simulink model "dynamical_model_extended"  (R2017b)
settings: Solver=ode4  StartTime=0.0  StopTime=3  FixedStep=dt  RelTol=1e-3
undefined symbols (not defined in the file or in its folder): alpha0, c1, c2, c3, d0, dq_0, g, m, p_true, q_0, r
libraries: dspinverses x2
(part 3 of 3)

== matlab function dynamical_model_extended/soft robotic manipulator dynamical model/Inertia matrix  ==
  data: q input; y output; m parameter; r parameter
function y = fcn(q,m,r)

l1 = q(1);
kappa_x1 = q(2);
kappa_y1 = q(3);

M = zeros(3,3);

% M(1,1) = (2.0*kappa_x1^2*l1*m*(kappa_x1^2 + kappa_y1^2)^(3/2) - 4.0*kappa_x1^4*m*sin(l1*(kappa_x1^2 + kappa_y1^2)^(1/2)) + 2.0*kappa_x1^4*l1*m*(kappa_x1^2 + kappa_y1^2)^(1/2) + 0.66666666666666666666666666666667*kappa_y1^4*l1^3*m*(kappa_x1^2 + kappa_y1^2)^(3/2) - 4.0*kappa_x1^2*kappa_y1^2*m*sin(l1*(kappa_x1^2 + kappa_y1^2)^(1/2)) + 2.0*kappa_x1^2*kappa_y1^2*l1*m*(kappa_x1^2 + kappa_y1^2)^(1/2) + (2/3)*kappa_x1^2*kappa_y1^2*l1^3*m*(kappa_x1^2 + kappa_y1^2)^(3/2))/(l1*(kappa_x1^2 + kappa_y1^2)^(7/2));
% M(1,2) =  -(1.0*kappa_x1*m*((kappa_x1^2 + kappa_y1^2)/kappa_x1^2)^(1/2)*(2.0*cos(l1*(kappa_x1^2 + kappa_y1^2)^(1/2))*(kappa_x1^2 + kappa_y1^2)^(1/2) - 2.0*(kappa_x1^2 + kappa_y1^2)^(1/2) + 2.0*kappa_x1^2*l1*sin(l1*(kappa_x1^2 + kappa_y1^2)^(1/2)) + 2.0*kappa_y1^2*l1*sin(l1*(kappa_x1^2 + kappa_y1^2)^(1/2)) - kappa_x1^2*l1^2*(kappa_x1^2 + kappa_y1^2)^(1/2) - kappa_y1^2*l1^2*(kappa_x1^2 + kappa_y1^2)^(1/2)))/(l1*(kappa_x1^2 + kappa_y1^2)^3);
% M(1,3) = 0;
% 
% M(2,1) = M(1,2);
% M(2,2) = (1.6e34*kappa_x1^4*l1*m + 1.2e34*kappa_y1^4*l1*m + 2.6666666666666666666666666666667e33*kappa_x1^6*l1^3*m + 2.6666666666666666666666666666667e33*kappa_x1^2*kappa_y1^4*l1^3*m + 5.3333333333333333333333333333333e33*kappa_x1^4*kappa_y1^2*l1^3*m + 666666666666666666666666666666677.0*kappa_x1^8*l1^3*m*r^2 - 3.2e34*kappa_x1^2*m*sin(l1*(kappa_x1^2 + kappa_y1^2)^(1/2))*(kappa_x1^2 + kappa_y1^2)^(1/2) - 1.6e34*kappa_y1^2*m*sin(l1*(kappa_x1^2 + kappa_y1^2)^(1/2))*(kappa_x1^2 + kappa_y1^2)^(1/2) + 1.6e34*kappa_x1^4*l1*m*cos(l1*(kappa_x1^2 + kappa_y1^2)^(1/2)) + 2.0e33*kappa_y1^2*m*sin(2.0*l1*(kappa_x1^2 + kappa_y1^2)^(1/2))*(kappa_x1^2 + kappa_y1^2)^(1/2) + 2.8e34*kappa_x1^2*kappa_y1^2*l1*m + 7.0e33*kappa_y1^6*l1*m*r^2 - 8.0e33*kappa_y1^2*m*r^2*sin(l1*(kappa_x1^2 + kappa_y1^2)^(1/2))*(kappa_x1^2 + kappa_y1^2)^(3/2) + 1.6e34*kappa_x1^2*kappa_y1^2*l1*m*cos(l1*(kappa_x1^2 + kappa_y1^2)^(1/2)) + 1.0e33*kappa_y1^2*m*r^2*sin(2.0*l1*(kappa_x1^2 + kappa_y1^2)^(1/2))*(kappa_x1^2 + kappa_y1^2)^(3/2) - 500000000000000000000000000000000.0*kappa_y1^4*m*r^2*sin(2.0*l1*(kappa_x1^2 + kappa_y1^2)^(1/2))*(kappa_x1^2 + kappa_y1^2)^(1/2) + 1.5e34*kappa_x1^2*kappa_y1^4*l1*m*r^2 + 8.0e33*kappa_x1^4*kappa_y1^2*l1*m*r^2 + 1.3333333333333333333333333333333e33*kappa_x1^2*kappa_y1^6*l1^3*m*r^2 + 3.3333333333333333333333333333333e33*kappa_x1^4*kappa_y1^4*l1^3*m*r^2 + 2.6666666666666666666666666666667e33*kappa_x1^6*kappa_y1^2*l1^3*m*r^2 - 4.0e33*kappa_x1^2*kappa_y1^2*m*r^2*sin(l1*(kappa_x1^2 + kappa_y1^2)^(1/2))*(kappa_x1^2 + kappa_y1^2)^(1/2) + 4.0e33*kappa_x1^2*kappa_y1^4*l1*m*r^2*cos(l1*(kappa_x1^2 + kappa_y1^2)^(1/2)) + 4.0e33*kappa_x1^4*kappa_y1^2*l1*m*r^2*cos(l1*(kappa_x1^2 + kappa_y1^2)^(1/2)) - 1.0e33*kappa_x1^2*kappa_y1^2*m*r^2*sin(2.0*l1*(kappa_x1^2 + kappa_y1^2)^(1/2))*(kappa_x1^2 + kappa_y1^2)^(1/2))/(4000000000000000000000000000000000*l1*(kappa_x1^2 + kappa_y1^2)^4);
% M(2,3) = (kappa_x1*kappa_y1*m*(1.0e33*kappa_x1^2*l1 - 500000000000000000000000000000000.0*sin(2.0*l1*(kappa_x1^2 + kappa_y1^2)^(1/2))*(kappa_x1^2 + kappa_y1^2)^(1/2) - 4.0e33*sin(l1*(kappa_x1^2 + kappa_y1^2)^(1/2))*(kappa_x1^2 + kappa_y1^2)^(1/2) + 1.0e33*kappa_y1^2*l1 + 666666666666666666666666666666677.0*kappa_x1^4*l1^3 + 666666666666666666666666666666677.0*kappa_y1^4*l1^3 + 2.0e33*r^2*sin(l1*(kappa_x1^2 + kappa_y1^2)^(1/2))*(kappa_x1^2 + kappa_y1^2)^(3/2) + 4.0e33*kappa_x1^2*l1*cos(l1*(kappa_x1^2 + kappa_y1^2)^(1/2)) + 4.0e33*kappa_y1^2*l1*cos(l1*(kappa_x1^2 + kappa_y1^2)^(1/2)) - 250000000000000000000000000000000.0*r^2*sin(2.0*l1*(kappa_x1^2 + kappa_y1^2)^(1/2))*(kappa_x1^2 + kappa_y1^2)^(3/2) - 2.0e33*kappa_x1^4*l1*r^2 - 1.75e33*kappa_y1^4*l1*r^2 + 1.3333333333333333333333333333333e33*kappa_x1^2*kappa_y1^2*l1^3 + 166666666666666666666666666666677.0*kappa_x1^6*l1^3*r^2 + 333333333333333333333333333333333.0*kappa_y1^6*l1^3*r^2 + 250000000000000000000000000000000.0*kappa_x1^2*r^2*sin(2.0*l1*(kappa_x1^2 + kappa_y1^2)^(1/2))*(kappa_x1^2 + kappa_y1^2)^(1/2) + 125000000000000000000000000000000.0*kappa_y1^2*r^2*sin(2.0*l1*(kappa_x1^2 + kappa_y1^2)^(1/2))*(kappa_x1^2 + kappa_y1^2)^(1/2) - 3.75e33*kappa_x1^2*kappa_y1^2*l1*r^2 + 833333333333333333333333333333333.0*kappa_x1^2*kappa_y1^4*l1^3*r^2 + 666666666666666666666666666666677.0*kappa_x1^4*kappa_y1^2*l1^3*r^2 + 500000000000000000000000000000000.0*kappa_x1^2*r^2*sin(l1*(kappa_x1^2 + kappa_y1^2)^(1/2))*(kappa_x1^2 + kappa_y1^2)^(1/2) - 500000000000000000000000000000000.0*kappa_y1^2*r^2*sin(l1*(kappa_x1^2 + kappa_y1^2)^(1/2))*(kappa_x1^2 + kappa_y1^2)^(1/2) - 500000000000000000000000000000000.0*kappa_x1^4*l1*r^2*cos(l1*(kappa_x1^2 + kappa_y1^2)^(1/2)) + 500000000000000000000000000000000.0*kappa_y1^4*l1*r^2*cos(l1*(kappa_x1^2 + kappa_y1^2)^(1/2))))/(1000000000000000000000000000000000*l1*(kappa_x1^2 + kappa_y1^2)^4);
% 
% M(3,1) = 0;
% M(3,2) = M(2,3);
% M(3,3) = (1.2e34*kappa_x1^4*l1*m + 1.6e34*kappa_y1^4*l1*m + 2.6666666666666666666666666666667e33*kappa_y1^6*l1^3*m + 5.3333333333333333333333333333333e33*kappa_x1^2*kappa_y1^4*l1^3*m + 2.6666666666666666666666666666667e33*kappa_x1^4*kappa_y1^2*l1^3*m + 1.3333333333333333333333333333333e33*kappa_y1^8*l1^3*m*r^2 - 1.6e34*kappa_x1^2*m*sin(l1*(kappa_x1^2 + kappa_y1^2)^(1/2))*(kappa_x1^2 + kappa_y1^2)^(1/2) - 3.2e34*kappa_y1^2*m*sin(l1*(kappa_x1^2 + kappa_y1^2)^(1/2))*(kappa_x1^2 + kappa_y1^2)^(1/2) + 1.6e34*kappa_y1^4*l1*m*cos(l1*(kappa_x1^2 + kappa_y1^2)^(1/2)) + 2.0e33*kappa_x1^2*m*sin(2.0*l1*(kappa_x1^2 + kappa_y1^2)^(1/2))*(kappa_x1^2 + kappa_y1^2)^(1/2) + 2.8e34*kappa_x1^2*kappa_y1^2*l1*m + 8.0e33*kappa_x1^6*l1*m*r^2 - 8.0e33*kappa_x1^2*m*r^2*sin(l1*(kappa_x1^2 + kappa_y1^2)^(1/2))*(kappa_x1^2 + kappa_y1^2)^(3/2) + 1.6e34*kappa_x1^2*kappa_y1^2*l1*m*cos(l1*(kappa_x1^2 + kappa_y1^2)^(1/2)) + 1.0e33*kappa_x1^2*m*r^2*sin(2.0*l1*(kappa_x1^2 + kappa_y1^2)^(1/2))*(kappa_x1^2 + kappa_y1^2)^(3/2) - 1.0e33*kappa_x1^4*m*r^2*sin(2.0*l1*(kappa_x1^2 + kappa_y1^2)^(1/2))*(kappa_x1^2 + kappa_y1^2)^(1/2) + 7.0e33*kappa_x1^2*kappa_y1^4*l1*m*r^2 + 1.5e34*kappa_x1^4*kappa_y1^2*l1*m*r^2 + 3.3333333333333333333333333333333e33*kappa_x1^2*kappa_y1^6*l1^3*m*r^2 + 2.6666666666666666666666666666667e33*kappa_x1^4*kappa_y1^4*l1^3*m*r^2 + 666666666666666666666666666666677.0*kappa_x1^6*kappa_y1^2*l1^3*m*r^2 + 4.0e33*kappa_x1^2*kappa_y1^2*m*r^2*sin(l1*(kappa_x1^2 + kappa_y1^2)^(1/2))*(kappa_x1^2 + kappa_y1^2)^(1/2) - 4.0e33*kappa_x1^2*kappa_y1^4*l1*m*r^2*cos(l1*(kappa_x1^2 + kappa_y1^2)^(1/2)) - 4.0e33*kappa_x1^4*kappa_y1^2*l1*m*r^2*cos(l1*(kappa_x1^2 + kappa_y1^2)^(1/2)) - 500000000000000000000000000000000.0*kappa_x1^2*kappa_y1^2*m*r^2*sin(2.0*l1*(kappa_x1^2 + kappa_y1^2)^(1/2))*(kappa_x1^2 + kappa_y1^2)^(1/2))/(4000000000000000000000000000000000*l1*(kappa_x1^2 + kappa_y1^2)^4);
%  
%  
M(1,1) = (m*(l1*(kappa_x1^2 + kappa_y1^2)^(3/2) - 4.0*kappa_x1^2*sin(l1*(kappa_x1^2 + kappa_y1^2)^(1/2)) - 4.0*kappa_y1^2*sin(l1*(kappa_x1^2 + kappa_y1^2)^(1/2)) + 3.0*kappa_x1^2*l1*(kappa_x1^2 + kappa_y1^2)^(1/2) + 3.0*kappa_y1^2*l1*(kappa_x1^2 + kappa_y1^2)^(1/2)))/(l1*(kappa_x1^2 + kappa_y1^2)^(5/2));
M(1,2) = -(2*kappa_x1*m*(2.0*l1*(kappa_x1^2 + kappa_y1^2)^(1/2) - 3.0*sin(l1*(kappa_x1^2 + kappa_y1^2)^(1/2)) + l1*cos(l1*(kappa_x1^2 + kappa_y1^2)^(1/2))*(kappa_x1^2 + kappa_y1^2)^(1/2)))/(l1*(kappa_x1^2 + kappa_y1^2)^(5/2));
M(1,3) = -(2*kappa_y1*m*(2.0*l1*(kappa_x1^2 + kappa_y1^2)^(1/2) - 3.0*sin(l1*(kappa_x1^2 + kappa_y1^2)^(1/2)) + l1*cos(l1*(kappa_x1^2 + kappa_y1^2)^(1/2))*(kappa_x1^2 + kappa_y1^2)^(1/2)))/(l1*(kappa_x1^2 + kappa_y1^2)^(5/2));

M(2,1) = -(2*kappa_x1*m*(2.0*l1*(kappa_x1^2 + kappa_y1^2)^(1/2) - 3.0*sin(l1*(kappa_x1^2 + kappa_y1^2)^(1/2)) + l1*cos(l1*(kappa_x1^2 + kappa_y1^2)^(1/2))*(kappa_x1^2 + kappa_y1^2)^(1/2)))/(l1*(kappa_x1^2 + kappa_y1^2)^(5/2));
M(2,2) = (0.5*kappa_y1^2*m*sin(2.0*l1*(kappa_x1^2 + kappa_y1^2)^(1/2)) - 4.0*kappa_y1^2*m*sin(l1*(kappa_x1^2 + kappa_y1^2)^(1/2)) - 8.0*kappa_x1^2*m*sin(l1*(kappa_x1^2 + kappa_y1^2)^(1/2)) + 3.0*l1*m*(kappa_x1^2 + kappa_y1^2)^(3/2) + 0.125*kappa_y1^4*m*r^2*sin(2.0*l1*(kappa_x1^2 + kappa_y1^2)^(1/2)) + kappa_x1^2*l1*m*(kappa_x1^2 + kappa_y1^2)^(1/2) + 0.66666666666666666666666666666667*kappa_x1^2*l1^3*m*(kappa_x1^2 + kappa_y1^2)^(3/2) - 2.0*kappa_y1^4*m*r^2*sin(l1*(kappa_x1^2 + kappa_y1^2)^(1/2)) + 0.125*kappa_x1^2*kappa_y1^2*m*r^2*sin(2.0*l1*(kappa_x1^2 + kappa_y1^2)^(1/2)) + 1.5*kappa_y1^2*l1*m*r^2*(kappa_x1^2 + kappa_y1^2)^(3/2) + 0.25*kappa_y1^4*l1*m*r^2*(kappa_x1^2 + kappa_y1^2)^(1/2) + 0.16666666666666666666666666666667*kappa_x1^4*l1^3*m*r^2*(kappa_x1^2 + kappa_y1^2)^(3/2) - 2.0*kappa_x1^2*kappa_y1^2*m*r^2*sin(l1*(kappa_x1^2 + kappa_y1^2)^(1/2)) + 4.0*kappa_x1^2*l1*m*cos(l1*(kappa_x1^2 + kappa_y1^2)^(1/2))*(kappa_x1^2 + kappa_y1^2)^(1/2) + 0.16666666666666666666666666666667*kappa_x1^2*kappa_y1^2*l1^3*m*r^2*(kappa_x1^2 + kappa_y1^2)^(3/2) + 0.25*kappa_x1^2*kappa_y1^2*l1*m*r^2*(kappa_x1^2 + kappa_y1^2)^(1/2))/(l1*(kappa_x1^2 + kappa_y1^2)^(7/2));
M(2,3) = -(2.5e-34*kappa_x1*kappa_y1*m*(1.6e34*sin(l1*(kappa_x1^2 + kappa_y1^2)^(1/2)) + 2.0e33*sin(2.0*l1*(kappa_x1^2 + kappa_y1^2)^(1/2)) - 4.0e33*l1*(kappa_x1^2 + kappa_y1^2)^(1/2) - 2.6666666666666666666666666666667e33*l1^3*(kappa_x1^2 + kappa_y1^2)^(3/2) - 8.0e33*kappa_x1^2*r^2*sin(l1*(kappa_x1^2 + kappa_y1^2)^(1/2)) - 8.0e33*kappa_y1^2*r^2*sin(l1*(kappa_x1^2 + kappa_y1^2)^(1/2)) - 1.6e34*l1*cos(l1*(kappa_x1^2 + kappa_y1^2)^(1/2))*(kappa_x1^2 + kappa_y1^2)^(1/2) + 500000000000000000000000000000000.0*kappa_x1^2*r^2*sin(2.0*l1*(kappa_x1^2 + kappa_y1^2)^(1/2)) + 500000000000000000000000000000000.0*kappa_y1^2*r^2*sin(2.0*l1*(kappa_x1^2 + kappa_y1^2)^(1/2)) + 6.0e33*l1*r^2*(kappa_x1^2 + kappa_y1^2)^(3/2) - 666666666666666666666666666666677.0*kappa_x1^2*l1^3*r^2*(kappa_x1^2 + kappa_y1^2)^(3/2) - 666666666666666666666666666666677.0*kappa_y1^2*l1^3*r^2*(kappa_x1^2 + kappa_y1^2)^(3/2) + 1.0e33*kappa_x1^2*l1*r^2*(kappa_x1^2 + kappa_y1^2)^(1/2) + 1.0e33*kappa_y1^2*l1*r^2*(kappa_x1^2 + kappa_y1^2)^(1/2)))/(l1*(kappa_x1^2 + kappa_y1^2)^(7/2));

M(3,1) = -(2*kappa_y1*m*(2.0*l1*(kappa_x1^2 + kappa_y1^2)^(1/2) - 3.0*sin(l1*(kappa_x1^2 + kappa_y1^2)^(1/2)) + l1*cos(l1*(kappa_x1^2 + kappa_y1^2)^(1/2))*(kappa_x1^2 + kappa_y1^2)^(1/2)))/(l1*(kappa_x1^2 + kappa_y1^2)^(5/2));
M(3,2) = -(2.5e-34*kappa_x1*kappa_y1*m*(1.6e34*sin(l1*(kappa_x1^2 + kappa_y1^2)^(1/2)) + 2.0e33*sin(2.0*l1*(kappa_x1^2 + kappa_y1^2)^(1/2)) - 4.0e33*l1*(kappa_x1^2 + kappa_y1^2)^(1/2) - 2.6666666666666666666666666666667e33*l1^3*(kappa_x1^2 + kappa_y1^2)^(3/2) - 8.0e33*kappa_x1^2*r^2*sin(l1*(kappa_x1^2 + kappa_y1^2)^(1/2)) - 8.0e33*kappa_y1^2*r^2*sin(l1*(kappa_x1^2 + kappa_y1^2)^(1/2)) - 1.6e34*l1*cos(l1*(kappa_x1^2 + kappa_y1^2)^(1/2))*(kappa_x1^2 + kappa_y1^2)^(1/2) + 500000000000000000000000000000000.0*kappa_x1^2*r^2*sin(2.0*l1*(kappa_x1^2 + kappa_y1^2)^(1/2)) + 500000000000000000000000000000000.0*kappa_y1^2*r^2*sin(2.0*l1*(kappa_x1^2 + kappa_y1^2)^(1/2)) + 6.0e33*l1*r^2*(kappa_x1^2 + kappa_y1^2)^(3/2) - 666666666666666666666666666666677.0*kappa_x1^2*l1^3*r^2*(kappa_x1^2 + kappa_y1^2)^(3/2) - 666666666666666666666666666666677.0*kappa_y1^2*l1^3*r^2*(kappa_x1^2 + kappa_y1^2)^(3/2) + 1.0e33*kappa_x1^2*l1*r^2*(kappa_x1^2 + kappa_y1^2)^(1/2) + 1.0e33*kappa_y1^2*l1*r^2*(kappa_x1^2 + kappa_y1^2)^(1/2)))/(l1*(kappa_x1^2 + kappa_y1^2)^(7/2));
M(3,3) = (0.5*kappa_x1^2*m*sin(2.0*l1*(kappa_x1^2 + kappa_y1^2)^(1/2)) - 8.0*kappa_y1^2*m*sin(l1*(kappa_x1^2 + kappa_y1^2)^(1/2)) - 4.0*kappa_x1^2*m*sin(l1*(kappa_x1^2 + kappa_y1^2)^(1/2)) + 3.0*l1*m*(kappa_x1^2 + kappa_y1^2)^(3/2) + 0.125*kappa_x1^4*m*r^2*sin(2.0*l1*(kappa_x1^2 + kappa_y1^2)^(1/2)) + kappa_y1^2*l1*m*(kappa_x1^2 + kappa_y1^2)^(1/2) + 0.66666666666666666666666666666667*kappa_y1^2*l1^3*m*(kappa_x1^2 + kappa_y1^2)^(3/2) - 2.0*kappa_x1^4*m*r^2*sin(l1*(kappa_x1^2 + kappa_y1^2)^(1/2)) + 0.125*kappa_x1^2*kappa_y1^2*m*r^2*sin(2.0*l1*(kappa_x1^2 + kappa_y1^2)^(1/2)) + 1.5*kappa_x1^2*l1*m*r^2*(kappa_x1^2 + kappa_y1^2)^(3/2) + 0.25*kappa_x1^4*l1*m*r^2*(kappa_x1^2 + kappa_y1^2)^(1/2) + 0.16666666666666666666666666666667*kappa_y1^4*l1^3*m*r^2*(kappa_x1^2 + kappa_y1^2)^(3/2) - 2.0*kappa_x1^2*kappa_y1^2*m*r^2*sin(l1*(kappa_x1^2 + kappa_y1^2)^(1/2)) + 4.0*kappa_y1^2*l1*m*cos(l1*(kappa_x1^2 + kappa_y1^2)^(1/2))*(kappa_x1^2 + kappa_y1^2)^(1/2) + 0.16666666666666666666666666666667*kappa_x1^2*kappa_y1^2*l1^3*m*r^2*(kappa_x1^2 + kappa_y1^2)^(3/2) + 0.25*kappa_x1^2*kappa_y1^2*l1*m*r^2*(kappa_x1^2 + kappa_y1^2)^(1/2))/(l1*(kappa_x1^2 + kappa_y1^2)^(7/2));
 

y = M;

== matlab function dynamical_model_extended/soft robotic manipulator dynamical model/Potential ==
  data: q input; p_true parameter; d0 parameter; y output; alpha0 parameter; g parameter; m parameter
function y = fcn(q, p_true, d0, alpha0, g, m)

l1 = q(1);
kappa_x1 = q(2);
kappa_y1 = q(3);

% b1 =  1.4670;
% b2 = -144.2928;
% b3 = 317.2625;
% 
% b4 =  0.0509;      
% b5 = -0.9967;
% b6 =  0.0554;

b1 = p_true(1);
b2 = p_true(2);
b3 = p_true(3);
b4 = p_true(4);
b5 = p_true(5);
b6 = p_true(6);

G = zeros(3,1);

G(1) = (g*m*sin(l1*(kappa_x1^2 + kappa_y1^2)^(1/2)))/(l1*(kappa_x1^2 + kappa_y1^2)^(1/2)) - (alpha0 - l1*(kappa_x1^2 + kappa_y1^2)^(1/2))*(kappa_x1^2 + kappa_y1^2)^(1/2)*(b6 + b4*b5 - b4*b5*tanh(b5*(alpha0 - l1*(kappa_x1^2 + kappa_y1^2)^(1/2)))^2) - (2*g*m*sin((l1*(kappa_x1^2 + kappa_y1^2)^(1/2))/2)^2)/(l1^2*(kappa_x1^2 + kappa_y1^2)) - (d0 - l1)*(b3 + b1*b2 - b1*b2*tanh(b2*(d0 - l1))^2);
G(2) = (g*kappa_x1*m*sin(l1*(kappa_x1^2 + kappa_y1^2)^(1/2)))/(kappa_x1^2 + kappa_y1^2)^(3/2) - (kappa_x1*l1*(alpha0 - l1*(kappa_x1^2 + kappa_y1^2)^(1/2))*(b6 + b4*b5 - b4*b5*tanh(b5*(alpha0 - l1*(kappa_x1^2 + kappa_y1^2)^(1/2)))^2))/(kappa_x1^2 + kappa_y1^2)^(1/2) - (4*g*kappa_x1*m*sin((l1*(kappa_x1^2 + kappa_y1^2)^(1/2))/2)^2)/(l1*(kappa_x1^2 + kappa_y1^2)^2);
G(3) = (g*kappa_y1*m*sin(l1*(kappa_x1^2 + kappa_y1^2)^(1/2)))/(kappa_x1^2 + kappa_y1^2)^(3/2) - (kappa_y1*l1*(alpha0 - l1*(kappa_x1^2 + kappa_y1^2)^(1/2))*(b6 + b4*b5 - b4*b5*tanh(b5*(alpha0 - l1*(kappa_x1^2 + kappa_y1^2)^(1/2)))^2))/(kappa_x1^2 + kappa_y1^2)^(1/2) - (4*g*kappa_y1*m*sin((l1*(kappa_x1^2 + kappa_y1^2)^(1/2))/2)^2)/(l1*(kappa_x1^2 + kappa_y1^2)^2);
 
y = G;

== matlab function dynamical_model_extended/soft robotic manipulator dynamical model/DIssipation  ==
  data: dq input; y output; c1 parameter; c2 parameter; c3 parameter
function y = fcn(dq,c1,c2,c3)

dl1 = dq(1);
dkappa_x1 = dq(2);
dkappa_y1 = dq(3);


D = zeros(3,1);

D(1) = c1*dl1;
D(2) = c2*dkappa_x1;
D(3) = c3*dkappa_y1;

y = D;

== matlab function dynamical_model_extended/Subsystem/Jacobian  ==
  data: q input; J output; Jv output; Jw output
function [J,Jv,Jw] = fcn(q)
L = q(1); k_x = q(2); k_y = q(3);

J = [ (k_x*sin(L*(k_x^2 + k_y^2)^(1/2)))/(k_x^2 + k_y^2)^(1/2), (2*k_x^2*(cos(L*(k_x^2 + k_y^2)^(1/2)) - 1))/(k_x^2 + k_y^2)^2 - (cos(L*(k_x^2 + k_y^2)^(1/2)) - 1)/(k_x^2 + k_y^2) + (L*k_x^2*sin(L*(k_x^2 + k_y^2)^(1/2)))/(k_x^2 + k_y^2)^(3/2),                                                  (2*k_x*k_y*(cos(L*(k_x^2 + k_y^2)^(1/2)) - 1))/(k_x^2 + k_y^2)^2 + (L*k_x*k_y*sin(L*(k_x^2 + k_y^2)^(1/2)))/(k_x^2 + k_y^2)^(3/2);
      (k_y*sin(L*(k_x^2 + k_y^2)^(1/2)))/(k_x^2 + k_y^2)^(1/2),                                                  (2*k_x*k_y*(cos(L*(k_x^2 + k_y^2)^(1/2)) - 1))/(k_x^2 + k_y^2)^2 + (L*k_x*k_y*sin(L*(k_x^2 + k_y^2)^(1/2)))/(k_x^2 + k_y^2)^(3/2), (2*k_y^2*(cos(L*(k_x^2 + k_y^2)^(1/2)) - 1))/(k_x^2 + k_y^2)^2 - (cos(L*(k_x^2 + k_y^2)^(1/2)) - 1)/(k_x^2 + k_y^2) + (L*k_y^2*sin(L*(k_x^2 + k_y^2)^(1/2)))/(k_x^2 + k_y^2)^(3/2);
                                  cos(L*(k_x^2 + k_y^2)^(1/2)),                                                                    (L*k_x*cos(L*(k_x^2 + k_y^2)^(1/2)))/(k_x^2 + k_y^2) - (k_x*sin(L*(k_x^2 + k_y^2)^(1/2)))/(k_x^2 + k_y^2)^(3/2),                                                                    (L*k_y*cos(L*(k_x^2 + k_y^2)^(1/2)))/(k_x^2 + k_y^2) - (k_y*sin(L*(k_x^2 + k_y^2)^(1/2)))/(k_x^2 + k_y^2)^(3/2);
                                         (k_x^2 + k_y^2)^(1/2),                                                                                                                                                      (L*k_x)/(k_x^2 + k_y^2)^(1/2),                                                                                                                                                      (L*k_y)/(k_x^2 + k_y^2)^(1/2);
                                                             0,                                                                                                                                                               -k_y/(k_x^2 + k_y^2),                                                                                                                                                                k_x/(k_x^2 + k_y^2);
                                                             0,                                                                                                                                                                                  0,                                                                                                                                                                                  0];
                                                         
Jv = J(1:3,:);
Jw = J(4:6,:);
end

== matlab function dynamical_model_extended/Subsystem/Inverse kinematics with Groëbner basis ==
  data: x input; q output; y input; z input
function q = pToq(x,y,z)
    coder.extrinsic('warning')

    if z < 0
            warning('z<0 so the result may be wrong');
    end
    
    %% Determining phi, k and l
    phi = atan2(y,x);
    k = 2*sqrt(x^2+y^2)/(x^2 + y^2 + z^2);
    if k < 10^-99
        l = z;
    else
        l = asin(z*k)/k;
    end
    
    %% Determine kx and ky from phi and k
    if -pi/2 < phi && phi < pi/2
        kx =  sqrt(k^2 / (1+(tan(phi))^2));
        ky = kx * tan(phi);
    elseif phi == pi/2 || phi == -pi/2
        kx = 0;
        ky = k;
    else
        kx = -sqrt(k^2 / (1+(tan(phi))^2));
        ky = kx * tan(phi);
    end

    q = [l; kx; ky];
end

== matlab function dynamical_model_extended/MATLAB Function5 ==
  data: L input; kx input; p output; ky input
function p = qTop(L,kx,ky)
    k = sqrt(kx^2 + ky^2);
    phi = atan2(ky,kx);

    p = 1/k * [(1-cos(L*k))*cos(phi);
               (1-cos(L*k))*sin(phi);
                  sin(L*k)           ];
    
end
